simulink model "lbr4p_joint_impctrl_test"  (Simulink 9.0)
settings: Solver=ode4  StartTime=0.0  StopTime=2.0  FixedStep=1e-4  RelTol=1e-3  EnableMultiTasking=on
values from neighbouring files (symbols this model uses):
  B = 0*B    [lbr4p_joint_impctrl_test_start.m]
  D = 0.7*eye(NJ)    [lbr4p_joint_impctrl_test_start.m]
  F_ext_noise = 2.3    [lbr4p_joint_impctrl_test_start.m]
  F_ext_noise_seed = 0    [lbr4p_joint_impctrl_test_start.m]
  F_ext_noise_switch = 0    [lbr4p_joint_impctrl_test_start.m]
  g_base = [0;0;-9.81]    [lbr4p_joint_impctrl_test_start.m]
  g_noise = 2e-4    (= 0.0002)    [lbr4p_joint_impctrl_test_start.m]
  g_noise_seed = 0    [lbr4p_joint_impctrl_test_start.m]
  g_noise_switch = 0    [lbr4p_joint_impctrl_test_start.m]
  K_ext_o = 0    [lbr4p_joint_impctrl_test_start.m]
  K_fri_o = 0    [lbr4p_joint_impctrl_test_start.m]
  q_noise = 3.4e-4    (= 0.00034)    [lbr4p_joint_impctrl_test_start.m]
  q_noise_seed = 0    [lbr4p_joint_impctrl_test_start.m]
  q_noise_switch = 0    [lbr4p_joint_impctrl_test_start.m]
  qD_noise = 5.5e-2    (= 0.055)    [lbr4p_joint_impctrl_test_start.m]
  qD_noise_seed = 0    [lbr4p_joint_impctrl_test_start.m]
  qD_noise_switch = 0    [lbr4p_joint_impctrl_test_start.m]
  T = 0.0005    [lbr4p_joint_impctrl_test_start.m]
  tau_noise = 7.3e-2    (= 0.073)    [lbr4p_joint_impctrl_test_start.m]
  tau_noise_seed = 0    [lbr4p_joint_impctrl_test_start.m]
  tau_noise_switch = 0    [lbr4p_joint_impctrl_test_start.m]
undefined symbols (not defined in the file): K_d, K_ext_c, K_O, K_obs_c, K_qD_d, K_qDD_d, K_tau_a, K_tau_c, K_tau_D, K_tau_e, K_tau_f, K_tau_g, K_tau_K, K_tau_o, MPV_damp, MPV_model, pkin, qD_th, T1, tau_c, tau_th
libraries: lib_S7RRRRRRR1_dynamics x7, lbr4p_joint_impctrl_test_lib x3, lib_S7RRRRRRR1_kinematics x3, lib_joint_impctrl x3, lib_transformations x2
settings Model: LogicAnalyzerSignalOrdering=4d0e14aa-1e00-42a7-8a24-0439a9889711,180fdafb-ab13-41fd-b77a-28f0a7ec4ece,f67b1204-268e-4733-84ed-e30e3d28af7c  SuppressorTable=22 serialization::archive 11 0 6 0 0 0 11 0  Creator=knoechelmann  LastModifiedBy=schappler
settings DataIOCC: SaveFormat=StructureWithTime
settings DebuggingCC: SignalInfNanChecking=warning  SignalRangeChecking=warning  UnderspecifiedInitializationDetection=Simplified  MergeDetectMultiDrivingBlocksExec=error  SolverPrmCheckMsg=warning  MultiTaskRateTransMsg=warning  CheckMatrixSingularityMsg=warning  UnderSpecifiedDataTypeMsg=warning
settings GRTTargetCC: GeneratePreprocessorConditionals=Disable all
settings ConfigComp: CovSFcnEnable=off

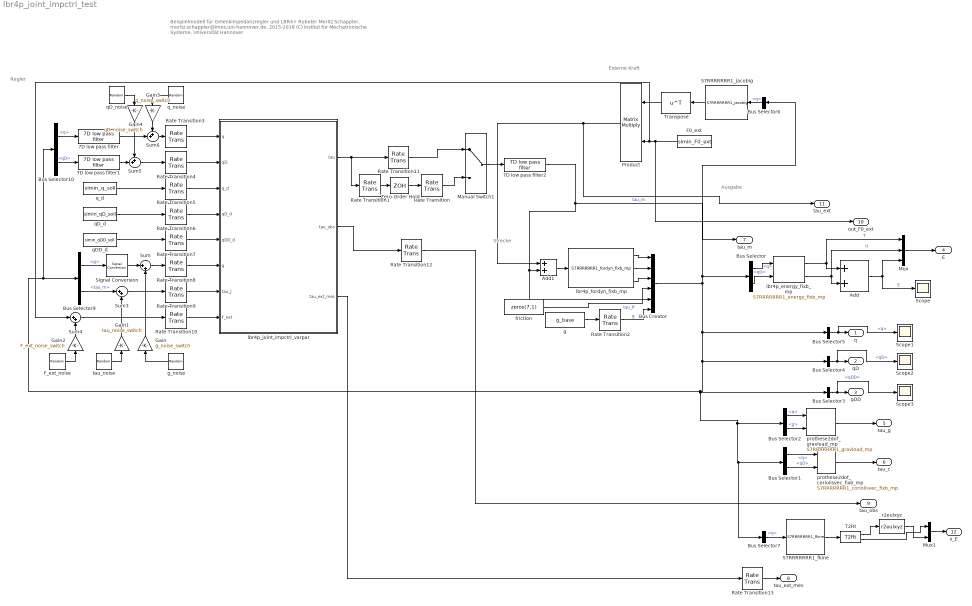
== system lbr4p_joint_impctrl_test ==
  note: Ausgabe
  note: Regler
  note: Externe Kraft
  note: Strecke
  note: Beispielmodell für Gelenkimpedanzregler und LBR4+ Roboter
      | Moritz Schappler, moritz.schappler@imes.uni-hannover.de, 2015-2018
      | (C) Institut für Mechatronische Systeme, Universität Hannover
  7D low pass filter : lbr4p_joint_impctrl_test_lib/7D low pass filter  f=T1_filter_input
  7D low pass filter1 : lbr4p_joint_impctrl_test_lib/7D low pass filter  f=T1_filter_input
  7D low pass filter2 : lbr4p_joint_impctrl_test_lib/7D low pass filter  f=T1_filter_input
  Add : Sum
  Add1 : Sum
  Bus Creator : BusCreator  Inputs='q','qD','qDD','tau_fr','tau_m','g'
  Bus Selector : BusSelector  OutputSignals=q,qD
  Bus Selector1 : BusSelector  OutputSignals=q,qD
  Bus Selector10 : BusSelector  OutputSignals=q,qD
  Bus Selector2 : BusSelector  OutputSignals=q,g
  Bus Selector3 : BusSelector  OutputSignals=qDD
  Bus Selector4 : BusSelector  OutputSignals=qD
  Bus Selector5 : BusSelector  OutputSignals=q
  Bus Selector6 : BusSelector  OutputSignals=q
  Bus Selector7 : BusSelector  OutputSignals=q
  Bus Selector9 : BusSelector  OutputSignals=g,tau_m
  F0_ext : FromWorkspace  VariableName=simin_F0_ext  SampleTime=0  Interpolate=off  OutputAfterFinalValue=Holding final value
  F_ext_noise : UniformRandomNumber  Minimum=-F_ext_noise  Maximum=F_ext_noise  Seed=F_ext_noise_seed  SampleTime=0
  Gain : Gain  Gain=g_noise_switch
  Gain1 : Gain  Gain=tau_noise_switch
  Gain2 : Gain  Gain=F_ext_noise_switch
  Gain3 : Gain  Gain=q_noise_switch
  Gain4 : Gain  Gain=qD_noise_switch
  Manual Switch1 : ManualSwitch
  Mux : Mux  Inputs=3
  Mux1 : Mux  Inputs=2
  Product : Product  Multiplication=Matrix(*)
  Rate Transition{,1..13} (14 alike) : RateTransition
  S7RRRRRRR1_fkine : lib_S7RRRRRRR1_kinematics/S7RRRRRRR1_fkine  pkin=pkin  iL=7
  S7RRRRRRR1_jacobig : lib_S7RRRRRRR1_kinematics/S7RRRRRRR1_jacobig  pkin=pkin  iL=7  r_i_i_C=zeros(3,1)
  Scope{,1..3} (4 alike) : Scope
  Signal Conversion : SignalConversion  OverrideOpt=off
  Sum : Sum  Inputs=|++
  Sum3 : Sum  Inputs=|++
  Sum4 : Sum  Inputs=|++
  Sum5 : Sum  Inputs=++|
  Sum6 : Sum  Inputs=++|
  T2Rt : lib_transformations/T2Rt
  Transpose : Math  Operator=transpose  SaturateOnIntegerOverflow=on
  Zero-Order Hold : ZeroOrderHold  SampleTime=0.001
  friction : Constant  Value=zeros(7,1)
  g : Constant  Value=g_base
  g_noise : UniformRandomNumber  Minimum=-g_noise  Maximum=g_noise  Seed=g_noise_seed  SampleTime=0
  lbr4p_energy_fixb_mp : lib_S7RRRRRRR1_dynamics/S7RRRRRRR1_energy_fixb_mp  pkin=pkin  MPV=MPV_plant  g_base=g_base
  lbr4p_fordyn_fixb_mp : lib_S7RRRRRRR1_dynamics/S7RRRRRRR1_fordyn_fixb_mp  q_t0=q_t0  qD_t0=qD_t0  g_base=g_base  pkin=pkin  MPV=MPV_plant
  lbr4p_joint_impctrl_varpar : Subsystem  TreatAsAtomicUnit=on  SystemSampleTime=T  mask(Atlas Joint Impedance Controller){K_d=K_d, D=D, K_tau_g=K_tau_g, K_tau_c=K_tau_c, K_tau_K=K_tau_K, K_tau_D=K_tau_D, K_tau_a=K_tau_a, K_tau_f=K_tau_f, K_tau_e=K_tau_e, K_tau_o=K_tau_o, K_qD_d=K_qD_d, K_qDD_d=K_qDD_d, K_ext_c=K_ext_c, K_obs_c=K_obs_c, K_fri_o=K_fri_o, K_ext_o=K_ext_o, MPV_damp=MPV_damp, MPV_model=MPV_model, pkin=pkin, tau_c=tau_c, B=B, qD_th=qD_th, tau_th=tau_th, K_O=K_O, T=T, T1=T1}
      mask prompts: K_d "K_d (desired stiffness)"; D "D (diagonal matrix with desired damping coefficients)"; K_tau_g "K_tau_g (gain of gravity compensation)"; K_tau_c "K_tau_c (gain of corriolis- and inertia compensation)"; K_tau_K "K_tau_K (gain of stiffness component)"; K_tau_D "K_tau_D (gain of damping component)"; K_tau_a "K_tau_a (gain of acceleration component)"; K_tau_f "K_tau_f (gain of model based friction compensation)"; K_tau_e "K_tau_e (gain of compensation of external torque measurd via hand sensor)"; K_tau_o "K_tau_o (gain of compensation of disturbance observer torques)"; K_qD_d "K_qD_d (gain of desired velocity)"; K_qDD_d "K_qDD_d (gain of desired acceleration)"; K_ext_c "K_ext_c (input gain to deside, wether to trigger friction compensation via the measured external torque)"; K_obs_c "K_obs_c (input gain to deside, wether to trigger friction compensation via the observed torque)"; K_fri_o "K_fri_o (input gain of friction model torques for observer)"; K_ext_o "K_ext_o (input gain of external torque for observer)"; MPV_damp "MPV_damp (base parameter vector for damping calculation)"; MPV_model "MPV_model (base parameter vector for dynamic model calculation)"; pkin "pkin (Kinematic Parameters)"; tau_c "tau_c (vector with coulomb friction momentums for all joints)"; B "B (vector with viscous friction coefficients of all joints)"; qD_th "qD_th (vector with theshold velocities for stiction)"; tau_th "tau_th (vector with kick-in momentums for stiction compensation)"; K_O "K_O (friction observer gain)"; T "T (sample time (important for friction observer))"; T1 "T1 (low pass filter time constant for inertia matrix)"
      mask help:
      | Hardware dependent full impedance controller block with matrix
      | squareroot damping design for the atlas robot. For a better
      | testing, all partial momentums can be individually scaled.
      | Coulomb-, viscous friction and Stribeck stiction is taken into
      | account for friction compensation.
  prothese2dof_coriolisvec_fixb_mp : lib_S7RRRRRRR1_dynamics/S7RRRRRRR1_coriolisvec_fixb_mp  pkin=pkin  MPV=MPV_plant
  prothese2dof_gravload_mp : lib_S7RRRRRRR1_dynamics/S7RRRRRRR1_gravload_mp  pkin=pkin  MPV=MPV_plant
  qDD_d : FromWorkspace  VariableName=simin_qDD_soll  SampleTime=0  OutputAfterFinalValue=Holding final value
  qD_d : FromWorkspace  VariableName=simin_qD_soll  SampleTime=0  OutputAfterFinalValue=Holding final value
  qD_noise : UniformRandomNumber  Minimum=-qD_noise  Maximum=qD_noise  Seed=qD_noise_seed  SampleTime=0
  q_d : FromWorkspace  VariableName=simin_q_soll  SampleTime=0  OutputAfterFinalValue=Holding final value
  q_noise : UniformRandomNumber  Minimum=-q_noise  Maximum=q_noise  Seed=q_noise_seed  SampleTime=0
  r2eulxyz : lib_transformations/r2eulxyz
  tau_noise : UniformRandomNumber  Minimum=-tau_noise  Maximum=tau_noise  Seed=tau_noise_seed  SampleTime=0
  q : Outport  PortDimensions=7
  qD : Outport  Port=2  PortDimensions=7
  qDD : Outport  Port=3  PortDimensions=7
  E : Outport  Port=4
  tau_g : Outport  Port=5  PortDimensions=7
  tau_c : Outport  Port=6  PortDimensions=7
  tau_m : Outport  Port=7
  tau_ext_mes : Outport  Port=8  PortDimensions=7
  tau_obs : Outport  Port=9  PortDimensions=7
  out_F0_ext : Outport  Port=10
  tau_ext : Outport  Port=11  PortDimensions=7
  x_E : Outport  Port=12  PortDimensions=6
  wires:
  lbr4p_energy_fixb_mp/1 -> Add/1, Mux/1  "T"
  lbr4p_energy_fixb_mp/2 -> Add/2, Mux/2  "U"
  Add/1 -> Scope/1, Mux/3  "E"
  S7RRRRRRR1_jacobig/1 -> Transpose/1
  Product/1 -> tau_ext/1, Add1/1
  F0_ext/1 -> out_F0_ext/1, Sum4/1, Product/2
  prothese2dof_gravload_mp/1 -> tau_g/1
  prothese2dof_coriolisvec_fixb_mp/1 -> tau_c/1
  qD_d/1 -> Rate Transition6/1
  qDD_d/1 -> Rate Transition7/1
  q_d/1 -> Rate Transition5/1
  Manual Switch1/1 -> 7D low pass filter2/1
  lbr4p_joint_impctrl_varpar/1(tau) -> Rate Transition11/1, Rate Transition1/1
  Rate Transition1/1 -> Zero-Order Hold/1
  Zero-Order Hold/1 -> Rate Transition/1
  Rate Transition/1 -> Manual Switch1/2
  Transpose/1 -> Product/1
  lbr4p_fordyn_fixb_mp/1 -> Bus Creator/1
  lbr4p_fordyn_fixb_mp/2 -> Bus Creator/2
  lbr4p_fordyn_fixb_mp/3 -> Bus Creator/3
  Bus Selector/2 -> lbr4p_energy_fixb_mp/2  "<qD>"
  Bus Selector/1 -> lbr4p_energy_fixb_mp/1  "<q>"
  Bus Selector1/1 -> prothese2dof_coriolisvec_fixb_mp/1  "<q>"
  Bus Selector1/2 -> prothese2dof_coriolisvec_fixb_mp/2  "<qD>"
  Bus Selector2/1 -> prothese2dof_gravload_mp/1  "<q>"
  friction/1 -> Bus Creator/4  "tau_fr"
  g/1 -> Rate Transition2/1
  Rate Transition2/1 -> Bus Creator/6  "g"
  Bus Selector6/1 -> S7RRRRRRR1_jacobig/1  "<q>"
  Bus Selector5/1 -> Scope1/1, q/1  "<q>"
  Bus Selector4/1 -> Scope2/1, qD/1  "<qD>"
  Bus Selector3/1 -> Scope3/1, qDD/1  "<qDD>"
  Bus Selector2/2 -> prothese2dof_gravload_mp/2  "<g>"
  Bus Selector9/1 -> Signal Conversion/1  "<g>"
  Bus Selector10/1 -> 7D low pass filter/1  "<q>"
  Bus Selector10/2 -> 7D low pass filter1/1  "<qD>"
  7D low pass filter2/1 -> Bus Creator/5, Add1/2, tau_m/1  "tau_m"
  Rate Transition3/1 -> lbr4p_joint_impctrl_varpar/1(q)
  Rate Transition4/1 -> lbr4p_joint_impctrl_varpar/2(qD)
  Rate Transition5/1 -> lbr4p_joint_impctrl_varpar/3(q_d)
  Rate Transition6/1 -> lbr4p_joint_impctrl_varpar/4(qD_d)
  Rate Transition7/1 -> lbr4p_joint_impctrl_varpar/5(qDD_d)
  Rate Transition8/1 -> lbr4p_joint_impctrl_varpar/6(g)
  Rate Transition9/1 -> lbr4p_joint_impctrl_varpar/7(tau_J)
  Rate Transition10/1 -> lbr4p_joint_impctrl_varpar/8(F_ext)
  Rate Transition11/1 -> Manual Switch1/1
  Rate Transition12/1 -> tau_obs/1
  lbr4p_joint_impctrl_varpar/3(tau_ext_mes) -> Rate Transition13/1
  Mux/1 -> E/1
  Rate Transition13/1 -> tau_ext_mes/1
  Signal Conversion/1 -> Sum/1
  Sum/1 -> Rate Transition8/1
  g_noise/1 -> Gain/1
  Bus Selector9/2 -> Sum3/1  "<tau_m>"
  Sum3/1 -> Rate Transition9/1
  tau_noise/1 -> Gain1/1
  Sum4/1 -> Rate Transition10/1
  F_ext_noise/1 -> Gain2/1
  7D low pass filter1/1 -> Sum5/2
  Sum5/1 -> Rate Transition4/1
  7D low pass filter/1 -> Sum6/2
  Sum6/1 -> Rate Transition3/1
  q_noise/1 -> Gain3/1
  qD_noise/1 -> Gain4/1
  Gain/1 -> Sum/2
  Gain1/1 -> Sum3/2
  Gain2/1 -> Sum4/2
  Gain3/1 -> Sum6/1
  Gain4/1 -> Sum5/1
  lbr4p_joint_impctrl_varpar/2(tau_obs) -> Rate Transition12/1
  Add1/1 -> lbr4p_fordyn_fixb_mp/1
  S7RRRRRRR1_fkine/1 -> T2Rt/1
  T2Rt/1 -> r2eulxyz/1
  T2Rt/2 -> Mux1/1
  r2eulxyz/1 -> Mux1/2
  Bus Creator/1 -> Bus Selector/1, Bus Selector6/1, Bus Selector3/1, Bus Selector7/1, Bus Selector1/1, Bus Selector2/1, Bus Selector10/1, Bus Selector9/1, Bus Selector4/1, Bus Selector5/1
  Bus Selector7/1 -> S7RRRRRRR1_fkine/1  "<q>"
  Mux1/1 -> x_E/1

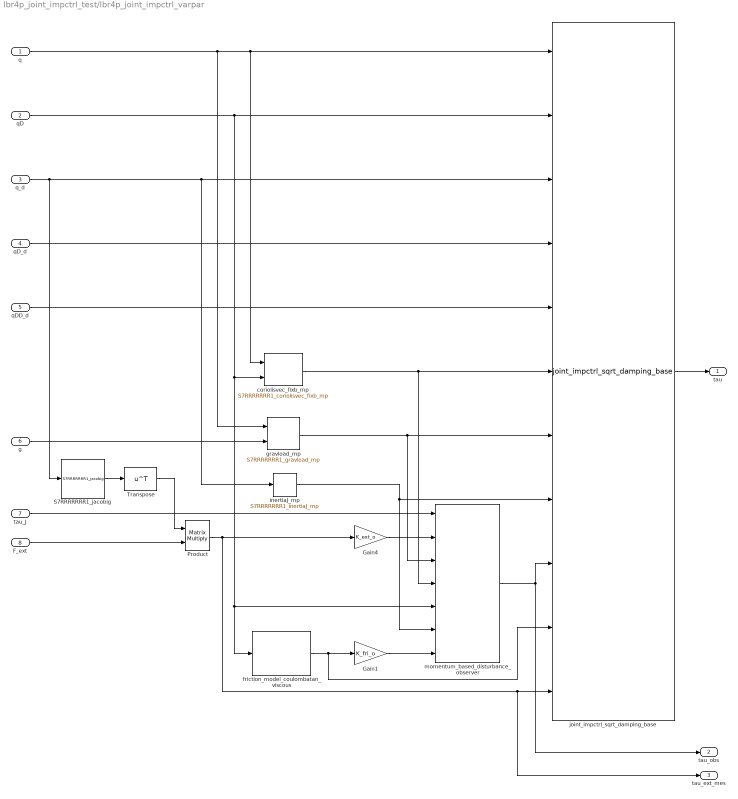
== system lbr4p_joint_impctrl_test/lbr4p_joint_impctrl_varpar ==
  q : Inport  OutDataTypeStr=double  PortDimensions=7
  qD : Inport  Port=2  OutDataTypeStr=double  PortDimensions=7
  q_d : Inport  Port=3  OutDataTypeStr=double  PortDimensions=7
  qD_d : Inport  Port=4  OutDataTypeStr=double  PortDimensions=7
  qDD_d : Inport  Port=5  OutDataTypeStr=double  PortDimensions=7
  g : Inport  Port=6  OutDataTypeStr=double  PortDimensions=3
  tau_J : Inport  Port=7  OutDataTypeStr=double  PortDimensions=7
  F_ext : Inport  Port=8  OutDataTypeStr=double  PortDimensions=6
  Gain1 : Gain  Gain=K_fri_o
  Gain4 : Gain  Gain=K_ext_o
  Product : Product  Multiplication=Matrix(*)
  S7RRRRRRR1_jacobig : lib_S7RRRRRRR1_kinematics/S7RRRRRRR1_jacobig  pkin=pkin  iL=7  r_i_i_C=zeros(3,1)
  Transpose : Math  Operator=transpose  SaturateOnIntegerOverflow=on
  coriolisvec_fixb_mp : lib_S7RRRRRRR1_dynamics/S7RRRRRRR1_coriolisvec_fixb_mp  pkin=pkin  MPV=MPV_model
  friction_model_coulombatan_viscous : lib_joint_impctrl/friction_model_coulombatan_viscous  tau_c=tau_c  B=B
  gravload_mp : lib_S7RRRRRRR1_dynamics/S7RRRRRRR1_gravload_mp  pkin=pkin  MPV=MPV_model
  inertiaJ_mp : lib_S7RRRRRRR1_dynamics/S7RRRRRRR1_inertiaJ_mp  pkin=pkin  MPV=MPV_damp
  joint_impctrl_sqrt_damping_base : lib_joint_impctrl/joint_impctrl_sqrt_damping_base  K_d=K_d  D=D  K_tau_g=K_tau_g  K_tau_c=K_tau_c  K_tau_K=K_tau_K  K_tau_D=K_tau_D  K_tau_a=K_tau_a  K_tau_f=K_tau_f  K_tau_e=K_tau_e  K_tau_o=K_tau_o  K_qD_d=K_qD_d  K_qDD_d=K_qDD_d  K_ext_c=K_ext_c  K_obs_c=K_obs_c  tau_c=tau_c  B=B  qD_th=qD_th  tau_th=tau_th
  momentum_based_disturbance_observer : lib_joint_impctrl/momentum_based_disturbance_observer  K_O=K_O  T=T  T1=T1  tau_out_max=30*ones(7,1)
  tau : Outport  OutDataTypeStr=double  PortDimensions=7
  tau_obs : Outport  Port=2  OutDataTypeStr=double  PortDimensions=7
  tau_ext_mes : Outport  Port=3  OutDataTypeStr=double  PortDimensions=7
  wires:
  Gain1/1 -> momentum_based_disturbance_observer/7
  Gain4/1 -> momentum_based_disturbance_observer/2
  friction_model_coulombatan_viscous/1 -> Gain1/1, joint_impctrl_sqrt_damping_base/10
  Product/1 -> Gain4/1, joint_impctrl_sqrt_damping_base/11, tau_ext_mes/1
  F_ext/1 -> Product/2
  Transpose/1 -> Product/1
  S7RRRRRRR1_jacobig/1 -> Transpose/1
  tau_J/1 -> momentum_based_disturbance_observer/1
  momentum_based_disturbance_observer/1 -> joint_impctrl_sqrt_damping_base/9, tau_obs/1
  g/1 -> gravload_mp/2
  qDD_d/1 -> joint_impctrl_sqrt_damping_base/5
  gravload_mp/1 -> joint_impctrl_sqrt_damping_base/7, momentum_based_disturbance_observer/3
  qD_d/1 -> joint_impctrl_sqrt_damping_base/4
  coriolisvec_fixb_mp/1 -> joint_impctrl_sqrt_damping_base/6, momentum_based_disturbance_observer/4
  q_d/1 -> S7RRRRRRR1_jacobig/1, joint_impctrl_sqrt_damping_base/3, inertiaJ_mp/1
  qD/1 -> coriolisvec_fixb_mp/2, momentum_based_disturbance_observer/5, friction_model_coulombatan_viscous/1, joint_impctrl_sqrt_damping_base/2
  q/1 -> joint_impctrl_sqrt_damping_base/1, coriolisvec_fixb_mp/1, gravload_mp/1
  inertiaJ_mp/1 -> joint_impctrl_sqrt_damping_base/8, momentum_based_disturbance_observer/6
  joint_impctrl_sqrt_damping_base/1 -> tau/1
